simulink model "Matfunct2"  (R2015a)
settings: Solver=ode4  StartTime=0.0  StopTime=5  FixedStep=1e-3  RelTol=1e-3
settings Model: Creator=Alumno  LastModifiedBy=HP
settings DebuggingCC: UnderspecifiedInitializationDetection=Classic  MergeDetectMultiDrivingBlocksExec=none  SolverPrmCheckMsg=warning

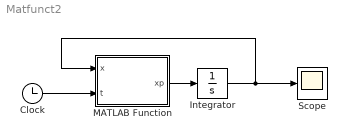
== system Matfunct2 ==
  Clock : Clock
  Integrator : Integrator  InitialCondition=[0 0]
  MATLAB Function : MATLAB Function  TreatAsAtomicUnit=on
  Scope : Scope
  wires:
  MATLAB Function/1(xp) -> Integrator/1
  Clock/1 -> MATLAB Function/2(t)
  Integrator/1 -> MATLAB Function/1(x), Scope/1

== matlab function Matfunct2/MATLAB Function ==
  data: x input; xp output; t input
function xp=fcn(x,t)
%#codegen
m=2;
k=1.5;
b=.2;
A=[0 1;-k/m -b/m];
B=[0;1/m];

u=3*t;
xp=A*x+B*u;
